simulink model "Torque2surface"  (R2018a)
settings: Solver=VariableStepAuto  StartTime=0.0  StopTime=5  RelTol=1e-3
settings Model: Creator=Ducted Fan  LastModifiedBy=Ducted Fan
settings SolverCC: ZeroCrossAlgorithm=Adaptive
settings DataIOCC: SaveOutput=off  SaveTime=off
settings DebuggingCC: MaxConsecutiveZCsMsg=none  MaskedZcDiagnostic=none  IgnoredZcDiagnostic=none

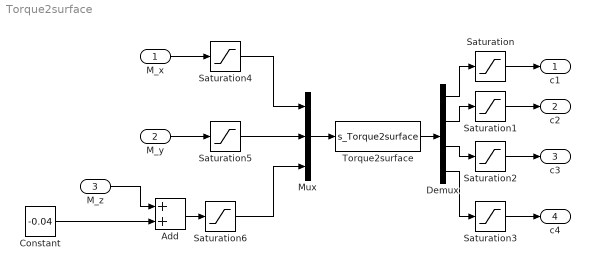
== system Torque2surface ==
  M_x : Inport  OutDataTypeStr=double  PortDimensions=1
  M_y : Inport  Port=2  OutDataTypeStr=double  PortDimensions=1
  M_z : Inport  Port=3  OutDataTypeStr=double  PortDimensions=1
  Add : Sum
  Constant : Constant  Value=-0.04
  Demux : Demux
  Mux : Mux  Inputs=3
  Saturation{,1..3} (4 alike) : Saturate  UpperLimit=0.34  LowerLimit=-0.34
  Saturation4 : Saturate  UpperLimit=0.349  LowerLimit=-0.349
  Saturation5 : Saturate  UpperLimit=0.349  LowerLimit=-0.349
  Saturation6 : Saturate  UpperLimit=0.349  LowerLimit=-0.349
  Torque2surface : S-Function  FunctionName=s_Torque2surface  SFunctionDeploymentMode=off  EnableBusSupport=off
  c1 : Outport  OutDataTypeStr=double  PortDimensions=1  SampleTime=0
  c2 : Outport  Port=2  OutDataTypeStr=double  PortDimensions=1  SampleTime=0
  c3 : Outport  Port=3  OutDataTypeStr=double  PortDimensions=1  SampleTime=0
  c4 : Outport  Port=4  OutDataTypeStr=double  PortDimensions=1  SampleTime=0
  wires:
  Mux/1 -> Torque2surface/1
  Torque2surface/1 -> Demux/1
  Saturation/1 -> c1/1
  Demux/1 -> Saturation/1
  Saturation1/1 -> c2/1
  Demux/2 -> Saturation1/1
  Saturation2/1 -> c3/1
  Demux/3 -> Saturation2/1
  Saturation3/1 -> c4/1
  Demux/4 -> Saturation3/1
  M_x/1 -> Saturation4/1
  M_y/1 -> Saturation5/1
  Saturation5/1 -> Mux/2
  Saturation4/1 -> Mux/1
  Saturation6/1 -> Mux/3
  Constant/1 -> Add/2
  M_z/1 -> Add/1
  Add/1 -> Saturation6/1
